simulink model "qbot2_data_collection"  (R2020a)
settings: Solver=ode1  StartTime=0.0  StopTime=D.t_end  FixedStep=0.02  RelTol=1e-3  EnableMultiTasking=on
StopFcn:
  | qbot2_post_DC
values from neighbouring files (symbols this model uses):
  D = rmfield(D, 'motion_plan')    [qbot2_motion_gen.m]
  x = rho.*cos(thetas)    [depth2xyz.m]
undefined symbols (not defined in the file or in its folder): HIL, Host, Kinect, qc_get_step_size, r
libraries: quarc_library x22, dspsigattribs x1, visiongeotforms x1
settings Model: SimulationMode=external  ExtModeTrigDuration=5000  Creator=icarus  LastModifiedBy=divad
settings SolverCC: PositivePriorityOrder=on
settings DataIOCC: MaxDataPoints=100000  SaveFormat=Array  ReturnWorkspaceOutputs=off
settings OptimizationCC: LifeSpan=inf
settings DebuggingCC: SolverPrmCheckMsg=warning  AllowSymbolicDim=off  SFUnexpectedBacktrackingDiag=warning  SFNoUnconditionalDefaultTransitionDiag=warning  SFExecutionAtInitializationDiag=none  ArithmeticOperatorsInVariantConditions=warning
settings HardwareCC: ProdBitPerPointer=32  ProdBitPerSizeT=32  ProdBitPerPtrDiffT=32  ProdLargestAtomicFloat=None  ProdIntDivRoundTo=Undefined  ProdEndianess=Unspecified  ProdWordSize=32  ProdHWDeviceType=32-bit Generic
settings ModelReferenceCC: PropagateSignalLabelsOutOfModel=off
settings SFSimCC: SimUseLocalCustomCode=off  CustomCodeUndefinedFunction=UseInterfaceOnly
settings RTWCC: Description=QUARC Linux DuoVero Target (QBall 2, QBot 2)  SystemTargetFile=quarc_linux_duovero.tlc  TemplateMakefile=quarc_linux_duovero_tmf  RTWUseLocalCustomCode=off
settings CodeAppCC: StateflowObjectComments=on
settings STFCustomTargetCC: TargetLibSuffix=.a  TargetPreCompLibLocation=C:\PROGRA~3\QUARC\lib\2020a\LINUX_~1\release  ConcurrentExecutionCompliant=on  GRTInterface=on  SystemTargetFile=quarc_linux_duovero.tlc
settings GRTTargetCC: TargetLibSuffix=.a  TargetPreCompLibLocation=C:\PROGRA~3\QUARC\lib\2020a\LINUX_~1\release  TargetLangStandard=C89/C90 (ANSI)  ParMdlRefBuildCompliant=off  CompOptLevelCompliant=off  CombineOutputUpdateFcns=off  MatFileLogging=off  CPPClassGenCompliant=off  GRTInterface=on  UseToolchainInfoCompliant=off  ExtMode=on  ExtModeMexFile=quarc_comm  ExtModeMexArgs='-w -d /tmp -uri %u'
settings ConfigComp: CovMetricSettings=dw  CovHTMLOptions=-sRT=1 -sVT=0 -aTS=1 -bRG=1 -bTC=1 -hTR=0 -nFC=0 -scm=1 -bcm=1 -xEv=0  CovHtmlReporting=on  CovSaveCumulativeToWorkspaceVar=on  CovSaveSingleToWorkspaceVar=on  CovExternalEMLEnable=off  CovSFcnEnable=off

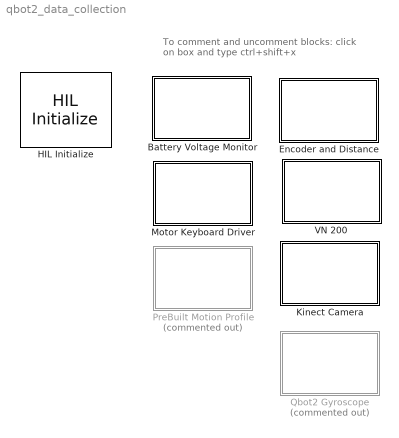
== system qbot2_data_collection ==
  note: To comment and uncomment blocks:
      | click on box and type ctrl+shift+x
  Battery Voltage Monitor : Subsystem
  Encoder and Distance : Subsystem
  HIL Initialize : quarc_library/Data Acquisition/Generic/Configuration/HIL Initialize  Priority=-99  object_name=HIL-1  board_type=qbot2  board_number=0  board_options=enc0_dir=0;enc0_filter=1;enc0_a=0;enc0_b=0;enc0_z=1;enc0_reload=0;enc1_dir=0;enc1_filter=1;enc1_a=0;enc1_b=0;enc1_z=1;enc1_reload=0;pwm0_immediate=0;pwm1_immediate=0;pwm2_immediate=0;pwm3_immediate=0;  exclusive=off  active=off  hardware_clocks=[]  clock_modes=[]  initial_clock_frequencies=[]  set_clock_params_at_start=off  set_clock_params_at_switch_in=off  set_clock_frequencies_at_start=off  set_clock_frequencies_at_switch_in=off  analog_input_channels=[0:9]  analog_input_configurations=[]  analog_input_maximums=[5 5 5 5 16.5 3.3 3.3 3.3 3.3]  analog_input_minimums=[0 0 0 0 0 0 0 0 0]  set_analog_input_params_at_start=off  set_analog_input_params_at_switch_in=off  analog_output_channels=[]  analog_output_maximums=[]  analog_output_minimums=[]  initial_analog_outputs=[]  final_analog_outputs=[]  watchdog_analog_outputs=[]  set_analog_output_params_at_start=off  set_analog_output_params_at_switch_in=off  set_analog_outputs_at_start=off  set_analog_outputs_at_switch_in=off  set_analog_outputs_at_terminate=off  set_analog_outputs_at_switch_out=off  set_analog_outputs_on_watchdog=off  digital_input_channels=[]  digital_output_channels=[]  digital_output_configuration=[]  initial_digital_outputs=[0]  final_digital_outputs=[0]  watchdog_digital_outputs=[0]  set_digital_output_params_at_start=off  set_digital_output_params_at_switch_in=off  set_digital_outputs_at_start=on  set_digital_outputs_at_switch_in=off  set_digital_outputs_at_terminate=on  set_digital_outputs_at_switch_out=off  set_digital_outputs_on_watchdog=on  encoder_channels=[0:3]  quadrature=[4]  encoder_filter_frequency=[]  initial_encoder_counts=[0]  set_encoder_params_at_start=on  set_encoder_params_at_switch_in=off  set_encoder_counts_at_start=on  set_encoder_counts_at_switch_in=off  pwm_channels=[0:3]  pwm_modes=[0]  pwm_frequency=[20e6/1024]  pwm_configuration=[0]  pwm_alignment=[0]  pwm_polarity=[1]  pwm_leading_deadband=[0]  pwm_trailing_deadband=[0]  initial_pwm_outputs=[0]  final_pwm_outputs=[0]  watchdog_pwm_outputs=[0]  set_pwm_params_at_start=on  set_pwm_params_at_switch_in=off  set_pwm_outputs_at_start=on  set_pwm_outputs_at_switch_in=off  set_pwm_outputs_at_terminate=on  set_pwm_outputs_at_switch_out=off  set_pwm_outputs_on_watchdog=on  other_output_channels=[2000:2001 14000 16000]  initial_other_outputs=[0 0 0 7]  final_other_outputs=[0 0 0 7]  watchdog_other_outputs=[]  set_other_outputs_at_start=on  set_other_outputs_at_switch_in=off  set_other_outputs_at_terminate=on  set_other_outputs_at_switch_out=off  set_other_outputs_on_watchdog=off
  Kinect Camera : Subsystem
  Motor Keyboard Driver : Subsystem
  PreBuilt Motion Profile : Subsystem  Commented=on
  Qbot2 Gyroscope : Subsystem  Commented=on
  VN 200 : Subsystem

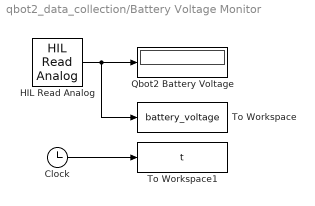
== system qbot2_data_collection/Battery Voltage Monitor ==
  Clock : Clock
  HIL Read Analog : quarc_library/Data Acquisition/Generic/Immediate I//O/HIL Read Analog  object_name=HIL-1  channels=[4]  sample_time=qc_get_step_size*100  active=on  vector_output=off
  Qbot2 Battery Voltage : Display
  To Workspace : ToWorkspace  VariableName=battery_voltage  SampleTime=-1
      settings: Save2DSignal=2-D array (concatenate along first dimension)
  To Workspace1 : ToWorkspace  VariableName=t  SampleTime=-1
      settings: Save2DSignal=2-D array (concatenate along first dimension)
  wires:
  HIL Read Analog/1 -> To Workspace/1, Qbot2 Battery Voltage/1
  Clock/1 -> To Workspace1/1

== system qbot2_data_collection/Encoder and Distance ==
  HIL Read Encoder : quarc_library/Data Acquisition/Generic/Immediate I//O/HIL Read Encoder  object_name=HIL-1  channels=[2:3]  sample_time=qc_get_step_size  active=on  vector_output=on  data_type_mode=Inherit via back propagation  data_type=double
  To Workspace : ToWorkspace  VariableName=odo  SampleTime=-1
      settings: Save2DSignal=2-D array (concatenate along first dimension)
  cnt2dist : quarc_library/Devices/Quanser/Mobile Robots/QBot 2/QBot 2 Encoder Counts to Distance
      settings: SourceProductName=QUARC Targets
  wires:
  HIL Read Encoder/1 -> cnt2dist/1
  cnt2dist/1 -> To Workspace/1

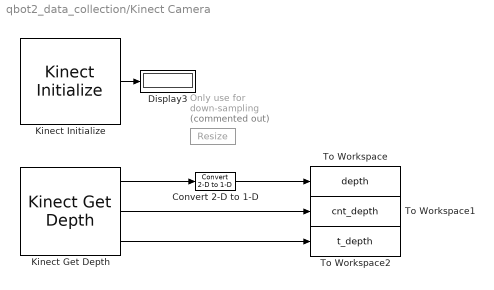
== system qbot2_data_collection/Kinect Camera ==
  Convert 2-D to 1-D : dspsigattribs/Convert 2-D to 1-D
      settings: SourceProductBaseCode=DS
  Display3 : Display
  Kinect Get Depth : quarc_library/Multimedia/Kinect Get Depth  object_name=Kinect-1  resolution=640 x 480  sample_time=1  show_player=off
      settings: SourceProductName=QUARC Targets
  Kinect Initialize : quarc_library/Multimedia/Kinect Initialize  object_name=Kinect-1  kinect_type=Kinect for XBox 360  identifier=0  sample_time=1  active=on
      settings: SourceProductName=QUARC Targets
  Only use for down-sampling : visiongeotforms/Resize  Commented=on  specify=Number of output rows and columns  rfactor=[200 150]  outCols=25  outRows=25  outRowsCols=[640/10 480/10]  interp_method=Nearest neighbor  antialias=off  useROI=off  roiFlag=off  roundingMode=Nearest  overflowMode=on  prodOutputMode=Binary point scaling  prodOutputWordLength=32  prodOutputFracLength=10
      settings: SourceProductBaseCode=VP
  To Workspace : ToWorkspace  VariableName=depth  SampleTime=-1
      settings: Save2DSignal=2-D array (concatenate along first dimension)
  To Workspace1 : ToWorkspace  VariableName=cnt_depth  SampleTime=-1
      settings: Save2DSignal=2-D array (concatenate along first dimension)
  To Workspace2 : ToWorkspace  VariableName=t_depth  SampleTime=-1
      settings: Save2DSignal=2-D array (concatenate along first dimension)
  wires:
  Kinect Initialize/1 -> Display3/1
  Kinect Get Depth/3 -> To Workspace2/1
  Kinect Get Depth/2 -> To Workspace1/1
  Convert 2-D to 1-D/1 -> To Workspace/1
  Kinect Get Depth/1 -> Convert 2-D to 1-D/1

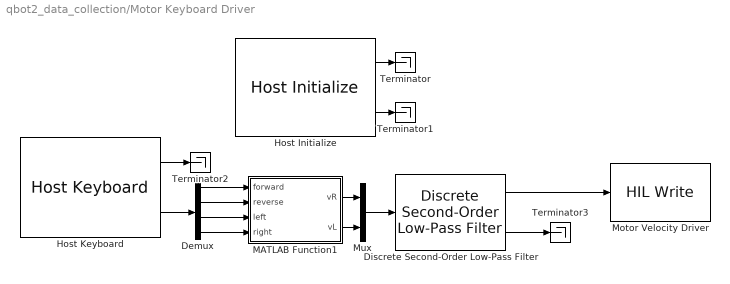
== system qbot2_data_collection/Motor Keyboard Driver ==
  Demux : Demux
  Discrete Second-Order Low-Pass Filter : quarc_library/Discrete/Discrete Second-Order Low-Pass Filter  params_source=Internal (dialog parameters)  input_width=2*pi*2.5  input_zeta=1  input_init=0  sample_time=qc_get_step_size
      settings: SourceProductName=QUARC Targets
  Host Initialize : quarc_library/Devices/Peripherals/Host/Host Initialize  object_name=Host-1  uri_source=Use external mode communications  uri=tcpip://localhost:18001  apply_uri_to_all_configs=on  send_buffer_size=1000  receive_buffer_size=1000  thread_priority=0  run_client=on  use_window=off  window_position=[]  sample_time=qc_get_step_size  active=on
      settings: SourceProductName=QUARC Targets
  Host Keyboard : quarc_library/Devices/Peripherals/Host/Host Keyboard  object_name=Host-1  virtual_key="[38  40  37  39]"  sample_time=qc_get_step_size  enabled=on  debug_mode=off
      settings: SourceProductName=QUARC Targets
  MATLAB Function1 : MATLAB Function  TreatAsAtomicUnit=on
  Motor Velocity Driver : quarc_library/Data Acquisition/Generic/Immediate I//O/HIL Write  object_name=HIL-1  analog_channels=[]  pwm_channels=[]  digital_channels=[]  other_channels=[2000:2001]  sample_time=-1  active=off  vector_input=on
  Mux : Mux  Inputs=2
  Terminator{,1..3} (4 alike) : Terminator
  wires:
  Host Initialize/1 -> Terminator/1
  Host Initialize/2 -> Terminator1/1
  MATLAB Function1/2(vL) -> Mux/2
  Host Keyboard/1 -> Terminator2/1
  Discrete Second-Order Low-Pass Filter/2 -> Terminator3/1
  Demux/4 -> MATLAB Function1/4(right)
  MATLAB Function1/1(vR) -> Mux/1
  Demux/2 -> MATLAB Function1/2(reverse)
  Demux/3 -> MATLAB Function1/3(left)
  Host Keyboard/2 -> Demux/1
  Mux/1 -> Discrete Second-Order Low-Pass Filter/1
  Discrete Second-Order Low-Pass Filter/1 -> Motor Velocity Driver/1
  Demux/1 -> MATLAB Function1/1(forward)

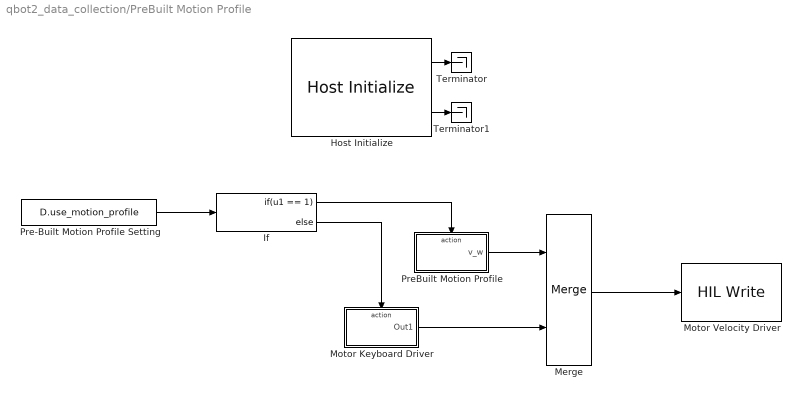
== system qbot2_data_collection/PreBuilt Motion Profile ==
  Host Initialize : quarc_library/Devices/Peripherals/Host/Host Initialize  object_name=Host-2  uri_source=Use external mode communications  uri=tcpip://localhost:18001  apply_uri_to_all_configs=on  send_buffer_size=1000  receive_buffer_size=1000  thread_priority=0  run_client=on  use_window=off  window_position=[]  sample_time=qc_get_step_size  active=on
      settings: SourceProductName=QUARC Targets
  If : If  IfExpression=u1 == 1
  Merge : Merge
  Motor Keyboard Driver : Subsystem  TreatAsAtomicUnit=on
  Motor Velocity Driver : quarc_library/Data Acquisition/Generic/Immediate I//O/HIL Write  object_name=HIL-1  analog_channels=[]  pwm_channels=[]  digital_channels=[]  other_channels=[2000:2001]  sample_time=-1  active=off  vector_input=on
  Pre-Built Motion Profile Setting : Constant  Value=D.use_motion_profile
  PreBuilt Motion Profile : Subsystem  TreatAsAtomicUnit=on
  Terminator : Terminator
  Terminator1 : Terminator
  wires:
  Host Initialize/1 -> Terminator/1
  Host Initialize/2 -> Terminator1/1
  Pre-Built Motion Profile Setting/1 -> If/1
  If/1 -> PreBuilt Motion Profile/Action
  If/2 -> Motor Keyboard Driver/Action
  PreBuilt Motion Profile/1(v_w) -> Merge/1
  Motor Keyboard Driver/1(Out1) -> Merge/2
  Merge/1 -> Motor Velocity Driver/1

== system qbot2_data_collection/Qbot2 Gyroscope ==
  HIL Read Other : quarc_library/Data Acquisition/Generic/Immediate I//O/HIL Read Other  object_name=HIL-1  channels=[3002]  sample_time=qc_get_step_size  active=on  vector_output=off
      settings: AttributesFormatString=(%<object_name>)  SourceProductName=QUARC Targets
  To Workspace : ToWorkspace  VariableName=gyro_qbot2  SaveFormat=Timeseries  SampleTime=-1
  wires:
  HIL Read Other/1 -> To Workspace/1

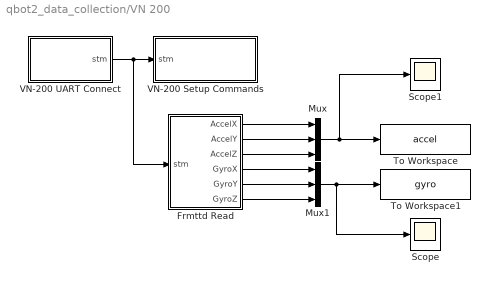
== system qbot2_data_collection/VN 200 ==
  Frmttd Read : Subsystem
  Mux : Mux  Inputs=3
  Mux1 : Mux  Inputs=3
  Scope : Scope
  Scope1 : Scope
  To Workspace : ToWorkspace  VariableName=accel  SampleTime=-1
      settings: Save2DSignal=2-D array (concatenate along first dimension)
  To Workspace1 : ToWorkspace  VariableName=gyro  SampleTime=-1
  VN-200 Setup Commands : Subsystem
  VN-200 UART Connect : Subsystem
  wires:
  Frmttd Read/1(AccelX) -> Mux/1
  Frmttd Read/2(AccelY) -> Mux/2
  Frmttd Read/3(AccelZ) -> Mux/3
  Frmttd Read/4(GyroX) -> Mux1/1
  Frmttd Read/6(GyroZ) -> Mux1/3
  Frmttd Read/5(GyroY) -> Mux1/2
  VN-200 UART Connect/1(stm) -> VN-200 Setup Commands/1(stm), Frmttd Read/1(stm)
  Mux1/1 -> Scope/1, To Workspace1/1
  Mux/1 -> Scope1/1, To Workspace/1

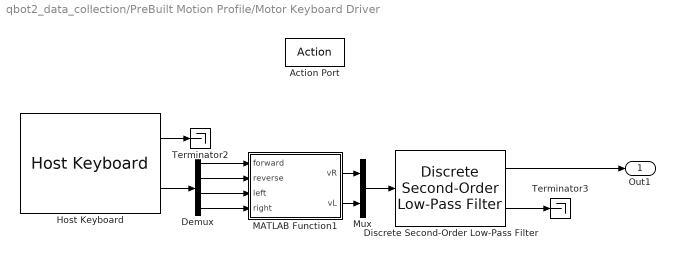
== system qbot2_data_collection/PreBuilt Motion Profile/Motor Keyboard Driver ==
  Action Port : ActionPort
  Demux : Demux
  Discrete Second-Order Low-Pass Filter : quarc_library/Discrete/Discrete Second-Order Low-Pass Filter  params_source=Internal (dialog parameters)  input_width=2*pi*2.5  input_zeta=1  input_init=0  sample_time=qc_get_step_size
      settings: SourceProductName=QUARC Targets
  Host Keyboard : quarc_library/Devices/Peripherals/Host/Host Keyboard  object_name=Host-2  virtual_key="[38  40  37  39]"  sample_time=qc_get_step_size  enabled=on  debug_mode=off
      settings: SourceProductName=QUARC Targets
  MATLAB Function1 : MATLAB Function  TreatAsAtomicUnit=on
  Mux : Mux  Inputs=2
  Terminator2 : Terminator
  Terminator3 : Terminator
  Out1 : Outport
  wires:
  Discrete Second-Order Low-Pass Filter/1 -> Out1/1
  MATLAB Function1/1(vR) -> Mux/1
  Demux/1 -> MATLAB Function1/1(forward)
  Mux/1 -> Discrete Second-Order Low-Pass Filter/1
  Demux/4 -> MATLAB Function1/4(right)
  Demux/2 -> MATLAB Function1/2(reverse)
  Discrete Second-Order Low-Pass Filter/2 -> Terminator3/1
  Demux/3 -> MATLAB Function1/3(left)
  Host Keyboard/1 -> Terminator2/1
  MATLAB Function1/2(vL) -> Mux/2
  Host Keyboard/2 -> Demux/1

== system qbot2_data_collection/PreBuilt Motion Profile/PreBuilt Motion Profile ==
  Action Port : ActionPort
  A better lookup table : MATLAB Function  TreatAsAtomicUnit=on
  v_w : Outport
  wires:
  A better lookup table/1(v_w) -> v_w/1

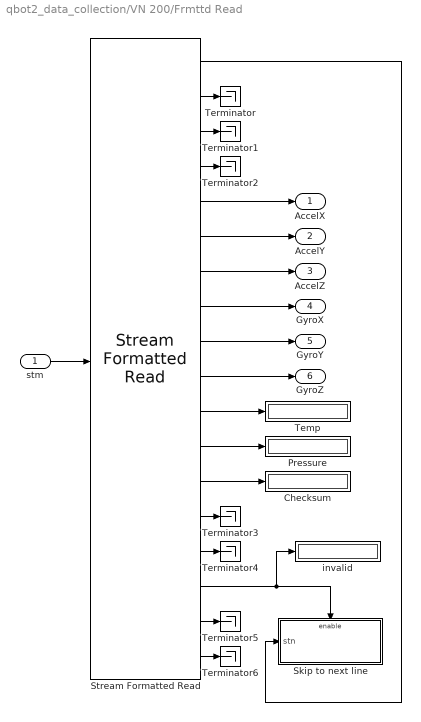
== system qbot2_data_collection/VN 200/Frmttd Read ==
  stm : Inport
  Checksum : Display
  Pressure : Display
  Skip to next line : Subsystem  TreatAsAtomicUnit=on
  Stream Formatted Read : quarc_library/Communications/Intermediate/Stream Formatted Read  format_string=$VNIMU,%f,%f,%f,%f,%f,%f,%f,%f,%f,%f,%f*%i\r  max_code_units=1000
      settings: SourceProductName=QUARC Targets
  Temp : Display
  Terminator{,1..6} (7 alike) : Terminator
  invalid : Display
  AccelX : Outport
  AccelY : Outport  Port=2
  AccelZ : Outport  Port=3
  GyroX : Outport  Port=4
  GyroY : Outport  Port=5
  GyroZ : Outport  Port=6
  wires:
  stm/1 -> Stream Formatted Read/1
  Stream Formatted Read/1 -> Skip to next line/1(stn)
  Stream Formatted Read/11 -> Temp/1
  Stream Formatted Read/12 -> Pressure/1
  Stream Formatted Read/13 -> Checksum/1
  Stream Formatted Read/16 -> invalid/1, Skip to next line/Enable
  Stream Formatted Read/5 -> AccelX/1
  Stream Formatted Read/8 -> GyroX/1
  Stream Formatted Read/9 -> GyroY/1
  Stream Formatted Read/10 -> GyroZ/1
  Stream Formatted Read/6 -> AccelY/1
  Stream Formatted Read/7 -> AccelZ/1
  Stream Formatted Read/2 -> Terminator/1
  Stream Formatted Read/3 -> Terminator1/1
  Stream Formatted Read/4 -> Terminator2/1
  Stream Formatted Read/14 -> Terminator3/1
  Stream Formatted Read/15 -> Terminator4/1
  Stream Formatted Read/17 -> Terminator5/1
  Stream Formatted Read/18 -> Terminator6/1

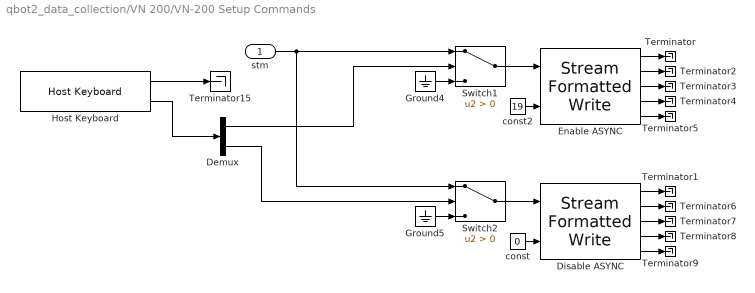
== system qbot2_data_collection/VN 200/VN-200 Setup Commands ==
  stm : Inport
  Demux : Demux  Outputs=2
  Disable ASYNC : quarc_library/Communications/Intermediate/Stream Formatted Write  format_string=$VNWRG,06,%i*XX\n  max_code_units=80  optimization=Minimizing latency
      settings: SourceProductName=QUARC Targets
  Enable ASYNC : quarc_library/Communications/Intermediate/Stream Formatted Write  format_string=$VNWRG,06,%i*XX\n  max_code_units=80  optimization=Minimizing latency
      settings: SourceProductName=QUARC Targets
  Ground4 : Ground
  Ground5 : Ground
  Host Keyboard : quarc_library/Devices/Peripherals/Host/Host Keyboard  object_name=Host-1  virtual_key="[69  68]"  sample_time=qc_get_step_size  enabled=on  debug_mode=off
      settings: SourceProductName=QUARC Targets
  Switch1 : Switch  Criteria=u2 > Threshold
  Switch2 : Switch  Criteria=u2 > Threshold
  Terminator{,1..9,15} (11 alike) : Terminator
  const : Constant  Value=0
  const2 : Constant  Value=19
  wires:
  const/1 -> Disable ASYNC/2
  const2/1 -> Enable ASYNC/2
  Enable ASYNC/1 -> Terminator/1
  Enable ASYNC/2 -> Terminator2/1
  Enable ASYNC/3 -> Terminator3/1
  Enable ASYNC/4 -> Terminator4/1
  Enable ASYNC/5 -> Terminator5/1
  Disable ASYNC/1 -> Terminator1/1
  Disable ASYNC/2 -> Terminator6/1
  Disable ASYNC/3 -> Terminator7/1
  Disable ASYNC/4 -> Terminator8/1
  Disable ASYNC/5 -> Terminator9/1
  Switch1/1 -> Enable ASYNC/1
  Switch2/1 -> Disable ASYNC/1
  Demux/1 -> Switch1/2
  Ground4/1 -> Switch1/3
  stm/1 -> Switch2/1, Switch1/1
  Ground5/1 -> Switch2/3
  Host Keyboard/1 -> Terminator15/1
  Host Keyboard/2 -> Demux/1
  Demux/2 -> Switch2/2

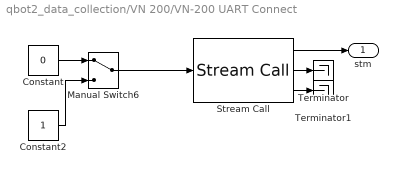
== system qbot2_data_collection/VN 200/VN-200 UART Connect ==
  Constant : Constant  Value=0
  Constant2 : Constant
  Manual Switch6 : ManualSwitch
  Stream Call : quarc_library/Communications/Intermediate/Stream Call  uri_source=Specify via dialog (do not evaluate)  uri=serial://localhost:1?baud='115200'  apply_uri_to_all_configs=on  send_buffer_size=80000  receive_buffer_size=80000  byte_order=little endian (Intel - LSB first)  sample_time=qc_get_step_size  non_blocking=on  active=on
      settings: AttributesFormatString="\"serial://localhost:1?baud='115200'\""  SourceProductName=QUARC Targets
  Terminator : Terminator
  Terminator1 : Terminator
  stm : Outport
  wires:
  Manual Switch6/1 -> Stream Call/1
  Constant/1 -> Manual Switch6/1
  Constant2/1 -> Manual Switch6/2
  Stream Call/1 -> stm/1
  Stream Call/2 -> Terminator/1
  Stream Call/3 -> Terminator1/1

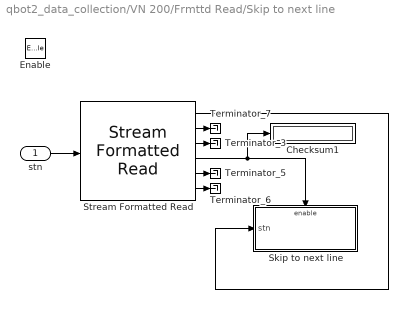
== system qbot2_data_collection/VN 200/Frmttd Read/Skip to next line ==
  stn : Inport
  Enable : EnablePort
  Checksum1 : Display
  Skip to next line : Subsystem  TreatAsAtomicUnit=on
  Stream Formatted Read : quarc_library/Communications/Intermediate/Stream Formatted Read  format_string=%*[^\r]  max_code_units=100
      settings: SourceProductName=QUARC Targets
  Terminator_{3,5..7} (4 alike) : Terminator
  wires:
  stn/1 -> Stream Formatted Read/1
  Stream Formatted Read/1 -> Skip to next line/1(stn)
  Stream Formatted Read/3 -> Terminator_3/1
  Stream Formatted Read/4 -> Checksum1/1, Skip to next line/Enable
  Stream Formatted Read/5 -> Terminator_5/1
  Stream Formatted Read/6 -> Terminator_6/1
  Stream Formatted Read/2 -> Terminator_7/1

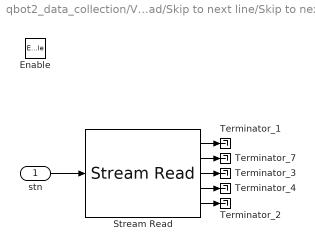
== system qbot2_data_collection/VN 200/Frmttd Read/Skip to next line/Skip to next line ==
  stn : Inport
  Enable : EnablePort
  Stream Read : quarc_library/Communications/Intermediate/Stream Read  data_type=Inherited via back propagation  type_expr=BusObject  num_elements=1  receive_dims=off
      settings: SourceProductName=QUARC Targets
  Terminator_{1..4,7} (5 alike) : Terminator
  wires:
  stn/1 -> Stream Read/1
  Stream Read/1 -> Terminator_1/1
  Stream Read/3 -> Terminator_3/1
  Stream Read/2 -> Terminator_7/1
  Stream Read/5 -> Terminator_2/1
  Stream Read/4 -> Terminator_4/1

== matlab function qbot2_data_collection/Motor Keyboard Driver/MATLAB Function1 ==
  data: forward input; vR output; vL output; reverse input; left input; right input
function [vR, vL] = fcn(forward, reverse, left, right)

persistent speed rot

maxspeed = 0.3;

if isempty(speed)
    speed = 0;
    rot = 0;
end

keystr = '0000';
if forward
    keystr(1) = '1';
end
if reverse
    keystr(2) = '1';
end
if left
    keystr(3) = '1';
end
if right
    keystr(4) = '1';
end

switch keystr
    case '1000'
        rot = 0;
        
        speed = maxspeed;
        vR = speed;
        vL = vR;
        
    case '0100'
        rot = 0;
        
        speed = -maxspeed;
        vR = speed;
        vL = vR;
        
    case '0010'
        rot = 1;
        
        speed = maxspeed/2;
        vR = speed;
        vL = -vR;
        
    case '0001'
        rot = 1;
        
        speed = -maxspeed/2;
        vR = speed;
        vL = -vR;
        
    otherwise
        if abs(speed) > 0
            speed = 0;
        end
            
        vR = speed;
        if rot
            vL = -speed;
        else
            vL = speed;
        end
end

== matlab function qbot2_data_collection/PreBuilt Motion Profile/Motor Keyboard Driver/MATLAB Function1 ==
  data: forward input; vR output; vL output; reverse input; left input; right input
function [vR, vL] = fcn(forward, reverse, left, right)

persistent speed rot

maxspeed = 0.3;

if isempty(speed)
    speed = 0;
    rot = 0;
end

keystr = '0000';
if forward
    keystr(1) = '1';
end
if reverse
    keystr(2) = '1';
end
if left
    keystr(3) = '1';
end
if right
    keystr(4) = '1';
end

switch keystr
    case '1000'
        rot = 0;
        
        speed = maxspeed;
        vR = speed;
        vL = vR;
        
    case '0100'
        rot = 0;
        
        speed = -maxspeed;
        vR = speed;
        vL = vR;
        
    case '0010'
        rot = 1;
        
        speed = maxspeed/2;
        vR = speed;
        vL = -vR;
        
    case '0001'
        rot = 1;
        
        speed = -maxspeed/2;
        vR = speed;
        vL = -vR;
        
    otherwise
        if abs(speed) > 0
            speed = 0;
        end
            
        vR = speed;
        if rot
            vL = -speed;
        else
            vL = speed;
        end
end

== matlab function qbot2_data_collection/PreBuilt Motion Profile/PreBuilt Motion Profile/A better lookup table ==
  data: v_w output double size=[2,1]; D parameter
function v_w  = prebuilt_motion_profile(D)

% provides values from look up table
persistent k

% Load New Index
if (isempty(k))
    k = 1;
end
    
% Isolate Values 
if (D.use_motion_profile == 1)
    v_w = D.v_cmds(:,k);
else
    v_w = zeros(2,1);
end

% Update Index
k = k + 1;
